simulink library "slx_LJM"  (R2024b)
settings: Solver=VariableStepAuto  StartTime=0.0  StopTime=10.0  RelTol=1e-3
libraries: simulink x3
settings Model: Creator=JulianBell  LastModifiedBy=GavinWilliamson
settings RTWCC: GPUComputeCapability=3.5

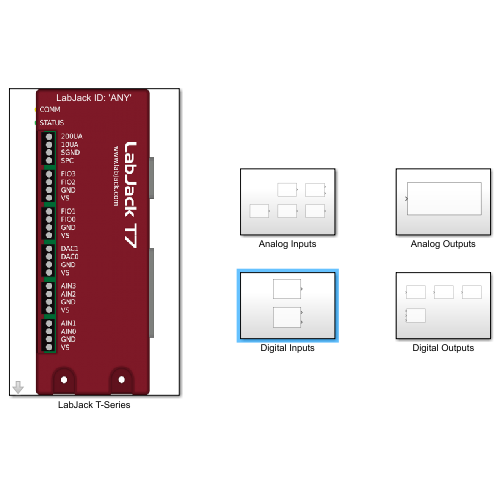
[thumbnail: Simulink's stored preview of the top-level diagram]
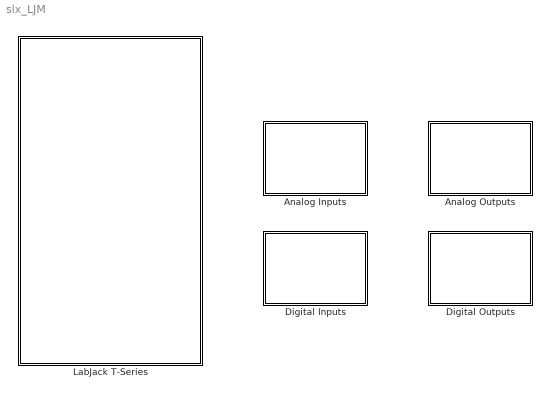
== system slx_LJM ==
  Analog Inputs : Subsystem
  Analog Outputs : Subsystem
  Digital Inputs : Subsystem
  Digital Outputs : Subsystem
  LabJack T-Series : Subsystem  mask{ljIdentifier='ANY', cnx_mth=USB, ljHandle=[]}
      mask prompts: ljIdentifier "LabJack Identifier [char]"; cnx_mth "Connection Method"; ljHandle "LabJack Handle"
      mask DialogControl DescGroupVar Prompt: LabJack T-Series
      mask DialogControl DescTextVar Prompt: This block is used to connect to a LabJack T4 or T7 device. Individual ports on the device can be configured, read, and written to by placing other blocks in the "slx_LJM" library within this block. This library link on this block must be disabled to place those block within this block.
      mask DialogControl Control4 Prompt: Once a simulation is stopped, the connection to the DIO ports are disabled, the LabJack clocks sare set to their default settings, and then the LabJack is disconnected. This is done through a Level-2 S-function block with the corresponding code in the "close_lbj.m" file.
      mask DialogControl Control2 Prompt: You can scan for any device that can be seen by inputting 'ANY' into the "LabJack Identifier" parameter. To connect to a specific device the serial number, IP address, or device name can be used. For more information please look at the documentaiton below.
      mask DialogControl Control3 Prompt: LabJack Connection Documentation
      mask Display:
      | image('ljT7.png');
      | idString = ["\color{White} LabJack ID: "+ get_param(gcb, 'ljIdentifier')];
      | text(0.5,0.98,idString,'horizontalAlignment','center','texmode','on');
      | 
      | %disp();

== system slx_LJM/Analog Inputs ==
  lj_AINRead : Subsystem  mask{ljPort="AIN0", ljRange=+/- 10V, Diff_Rd_SW=off, Diff_Rd="AIN1", ljHandle=32}
      mask prompts: ljPort "Port Name:"; ljRange "Voltage Range: (T7 Only)"; Diff_Rd_SW "Enable"; Diff_Rd "Negative Channel"; ljHandle "LabJack Handle"
      mask DialogControl DescGroupVar Prompt: AIN Read
      mask DialogControl DescTextVar Prompt: This block is used to read an analog input port. If using a T7 device the voltage range can be selected, and a differential reading can be chosen. If a differential reading is chosen, a valid negative channel must also be selected (typically the odd port for a pair of ports).  Voltage range selection and differential readings are not available on T4 devices.
      mask DialogControl Control4 Prompt: *For T4 devices the voltage range will be set to the default of the port (either +/- 10V or +/-2.5V) The parameter radio button do not effect the configuration.
      mask DialogControl Control3 Prompt: Differential Reading Documentation
      mask DialogControl Container3 Prompt: Differential Read (T7 Only)
      mask Display: disp(["AIN Read", "Port: "+ get_param(gcb, 'ljPort')]);
  lj_CurrentRead : Subsystem  mask{ljPort="AIN1", ljHandle=32, currentL=4, currentH=20, outputL=4, outputH=20}
      mask prompts: ljPort "Port Name:"; ljHandle "LabJack Handle"; currentL "Low Current (mA)"; currentH "High Current (mA)"; outputL "Low Output Value"; outputH "High Output Value"
      mask DialogControl DescGroupVar Prompt: Current Read
      mask DialogControl DescTextVar Prompt: This block is used for reading a current signal that is passed into the designated port using a LabJack current shunt. The block outputs the raw current reading as well as the scaled output based on the ranges set in the mask. The high and low output values correspond to the range of the sensor that you are reading.
      mask DialogControl Control2 Prompt: Current Shunt Documentation
      mask Display: disp(["Current Read", "Port: "+ get_param(gcb, 'ljPort')]);
  lj_RTDRead : Subsystem  mask{ljPort="AIN1", ljHandle=-1, rtdType=PT100, tempUnit=C, refResistance=1K}
      mask prompts: ljPort "Port Name:"; ljHandle "LabJack Handle"; rtdType "RTD Type"; tempUnit "Temperature Unit"; refResistance "Reference Resistance"
      mask DialogControl DescGroupVar Prompt: RTD Read
      mask DialogControl DescTextVar Prompt: This block is used to read an RTD.  The RTD type, temperature unit, and reference resistance can all be selected. This block assumes that exitation circuit #4 is being used, which is often implemented through the LabJack Resistance Tick.
      mask DialogControl RTD_doc Prompt: LabJack RTD Documentation
      mask DialogControl Ex_circ_4 Prompt: Excitation Circuit #4
      mask DialogControl res_tick Prompt: LabJack Resistance Tick
      mask Display: disp(["RTD Read", "Port: "+ get_param(gcb, 'ljPort')]);
  lj_ThermistorRead : Subsystem  mask{ljPort="AIN1", ljHandle=32, thermRes=1000, tempUnit=C, refResistance=10K, a=1.032e-3, b=2.387e-4, c=0, d=1.58e-7}
      mask prompts: ljPort "Port Name:"; ljHandle "LabJack Handle"; thermRes "Thermistor Resistance"; tempUnit "Temperature Unit"; refResistance "Reference Resistance"
      mask TypeOptions tempUnit: C | F | K
      mask DialogControl DescGroupVar Prompt: Thermistor Read
      mask DialogControl DescTextVar Prompt: This block is used to read a thermistor. This block assumes that exitation ciruit #4 is being used, which is often implemented thorugh a LabJack Resistance Tick. This block also configures the LabJack port to use the Steinhart-Hart equation. This configuartion can be altered in the mask's initialization code. The thermistor restistance, temperature unit, reference resistance, and Steinhart-Hart coefficients can all be set using the block's mask.
      mask DialogControl thermistor_doc Prompt: LabJack Thermistor Documentation
      mask DialogControl ex_circ_4 Prompt: Exitation Ciruit #4
      mask DialogControl res_tick Prompt: LabJack Resistance Tick
      mask DialogControl Container3 Prompt: Steinhart-Hart Coefficients
      mask Display: disp(["Thermistor Read", "Port: "+ get_param(gcb, 'ljPort')]);
  lj_ThermocoupleRead : Subsystem  mask{ljPort="AIN0", tempUnit=C, thermocoupleType=K, Diff_Rd_SW=off, Diff_Rd="AIN1", ljHandle=32}
      mask prompts: ljPort "Port Name:"; tempUnit "Temperature Units"; thermocoupleType "Thermocouple Type"; Diff_Rd_SW "Enable"; Diff_Rd "Negative Channel"; ljHandle "LabJack Handle"
      mask TypeOptions tempUnit: K | C | F
      mask TypeOptions thermocoupleType: E | J | K | R | T | S | N | B | C
      mask DialogControl DescGroupVar Prompt: Thermocouple Read
      mask DialogControl DescTextVar Prompt: This block is used to read a thermocouple. The thermocouple type and temperature units can be set in the block's mask. Differential reading can be enabled. If a differential reading is chosen, a valid negative channel must also be selected (typically the odd port for a pair of ports). This block only functions with T7 devices, not T4.
      mask DialogControl thermocouple_doc Prompt: LabJack Thermocouple Documentation
      mask DialogControl thermocouple_wir Prompt: LabJack Thermocouple Wiring
      mask DialogControl Container3 Prompt: Differential Read (T7 Only)
      mask Display: disp(["Thermocouple Read", "Port: "+ get_param(gcb, 'ljPort')]);

== system slx_LJM/Analog Outputs ==
  lj_DACWrite : Subsystem  mask{ljPort="DAC0", ljHandle=0}
      mask prompts: ljPort "LabJack DAC Port"; ljHandle "LabJack Handle"
      mask DialogControl DescGroupVar Prompt: DAC Write
      mask DialogControl DescTextVar Prompt: Block is used to output an analog signal throught the DAC ports. The typical output range for a T4/T7 device is 0-5V.
      mask DialogControl Control2 Prompt: LabJack DAC Documentation
      mask Display: disp(["DAC Write", "Port: "+ get_param(gcb, 'ljPort')]);

== system slx_LJM/Digital Inputs ==
  lj_DIORead : Subsystem  mask{ljPort="FIO1", ljHandle=[]}
      mask prompts: ljPort "Port ID"; ljHandle "LabJack Handle"
      mask DialogControl DescGroupVar Prompt: DIO Read
      mask DialogControl DescTextVar Prompt: This block is used to read a digital input port. An output value of 1 corresponds with a "high" value and an output value of 0 corresponds with a "low" value.
      mask DialogControl Control2 Prompt: LabJack Digital I/O Documentation
      mask Display: disp(["DIO Read", "Port: "+ get_param(gcb, 'ljPort')]);
  lj_FrequencyRead : Subsystem  mask{ljPort="DIO1", meas_typ=Rising-to-Rising Edge, ljClock=Clock 0 (32-bit), ljHandle=[]}
      mask prompts: ljPort "Port ID"; meas_typ "Measurement Type"; ljClock "Select LabJack Clock"; ljHandle "LabJack Handle"
      mask DialogControl DescGroupVar Prompt: Frequency Read
      mask DialogControl DescTextVar Prompt: This block is used to take a frequency reading of a diginal input port. The Port ID must be in the format "DIO#" so that the corresponding LabJack port can be properly configured. The measurement type and LabJack clock used to read frequency can also be selected. Caution should be used when selecting a LabJack clock to ensure there are no conflicts with other blocks in the LabJack. For more information, please see the documentation below.
      mask DialogControl Control2 Prompt: *It has been observed that the LabJack will occasionally read a period of 0 and a frequency of "nan" between valid reading of the correct frequency.
      mask DialogControl freq_in_data Prompt: LabJack Frequency In Datasheet
      mask DialogControl config_freq_in Prompt: Configuring & Reading Frequency
      mask DialogControl clock_web Prompt: LabJack Clock Source
      mask Display: disp(["Frequency Read", "Port: "+ get_param(gcb, 'ljPort')]);

== system slx_LJM/Digital Outputs ==
  lj_DACTickWrite : Subsystem  mask{ljPort="FIO0", ljHandle=2}
      mask prompts: ljPort "Port ID"; ljHandle "LabJack Handle"
      mask DialogControl DescGroupVar Prompt: DAC Tick Write
      mask DialogControl DescTextVar Prompt: This block is desinged to be used with a LabJack DAC to write a +/-10V signal out of a digital output port. This block will cause the LabJack matlab library to error if a DAC tick is not connected to the correct port.
      mask DialogControl Control2 Prompt: Labjack DAC Tick Documentation
      mask Display: disp(["DAC Tick Write", "Port: "+ get_param(gcb, 'ljPort')]);
  lj_DIOWrite : Subsystem  mask{ljPort="FIO0", defaultState=Low, ljHandle=2}
      mask prompts: ljPort "Port ID"; defaultState "Default Output State"; ljHandle "LabJack Handle"
      mask DialogControl DescGroupVar Prompt: DIO Write
      mask DialogControl DescTextVar Prompt: This block is used to write out of a digital output port. The default output state can be chosen. An input constant of 1 corresponds to a "high" value being written and an input constant of 0 corresponds with a "low" value being written.
      mask DialogControl Control2 Prompt: LabJack Digital I/O Documentation
      mask Display: disp(["DIO Write", "Port: "+ get_param(gcb, 'ljPort')]);
  lj_Heartbeat : Subsystem  mask{ljPort="FIO0", Simulink_step=1, ljHandle=2}
      mask prompts: ljPort "Port ID"; Simulink_step "Simulink Sample Time"; ljHandle "LabJack Handle"
      mask DialogControl DescGroupVar Prompt: Heartbeat
      mask DialogControl DescTextVar Prompt: This block is intended to be used as a watchdog to ensure that Simulink and the Labjack are still communicating properly. A 50% duty PWM is generated out of the specified port with the period that is passed into the input of the block. The sample time (step size) of the Simulink model must also be input into the mask parameters. The period input must be twice that of the Simulink sample time, and ideally 10x to ensure the most reliable performance of this block.
      mask Display: disp(["Heartbeat", "Port: "+ get_param(gcb, 'ljPort')]);
  lj_PWM : Subsystem  mask{ljPort="DIO0", defaultState=Low, ljClock=Clock 0 (32-bit), ljHandle=2}
      mask prompts: ljPort "Port ID"; defaultState "Default Output State"; ljClock "Select LabJack Clock"; ljHandle "LabJack Handle"
      mask DialogControl DescGroupVar Prompt: DIO PWM Write
      mask DialogControl DescTextVar Prompt: This block is used to write a PWM signal out of a DIO port. The portname should be in the format "DIO#" so that the port can be properly configured. The frequency, duty cycle, and enabling of the PWM is controlled by the block's input ports and can be updated while the simulatioin is running. A default output state can be chosen as well as the LabJack Clock that the PWM will use. Caution must be used when selecting which clock especially if multiple PWM write or read blocks are used in the same LabJack block. Please refer to the documentation below for addtional information.
      mask DialogControl pwm_data Prompt: LabJack PWM Out Datasheet
      mask DialogControl pwm_config Prompt: Configuring a PWM Output
      mask DialogControl clock_web Prompt: LabJack Clock Source
      mask Display: disp(["DIO PWM Write", "Port: "+ get_param(gcb, 'ljPort')]);

== system slx_LJM/LabJack T-Series ==
  Constant : Constant  Value=ljHandle
  Display : Display
  Level-2 MATLAB S-Function : M-S-Function  FunctionName=close_lbj
      mask DialogControl DescGroupVar Prompt: close_lbj
      mask DialogControl DescTextVar Prompt: Level 2 S-Function
      mask DialogControl Control2 Prompt: Block takes the input of the Labjack Handle as an int32 signal, and outputs the handle as a int 32 signal. Block closes connection to the LabJack when a simulation is stopped.
  wires:
  Constant/1 -> Level-2 MATLAB S-Function/1
  Level-2 MATLAB S-Function/1 -> Display/1

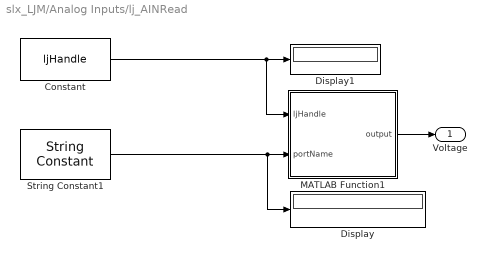
== system slx_LJM/Analog Inputs/lj_AINRead ==
  Constant : Constant  Value=ljHandle
  Display : Display
  Display1 : Display
  MATLAB Function1 : MATLAB Function  TreatAsAtomicUnit=on
  String Constant1 : StringConstant  String=ljPort
  Voltage : Outport
  wires:
  Constant/1 -> Display1/1, MATLAB Function1/1(ljHandle)
  MATLAB Function1/1(output) -> Voltage/1
  String Constant1/1 -> MATLAB Function1/2(portName), Display/1

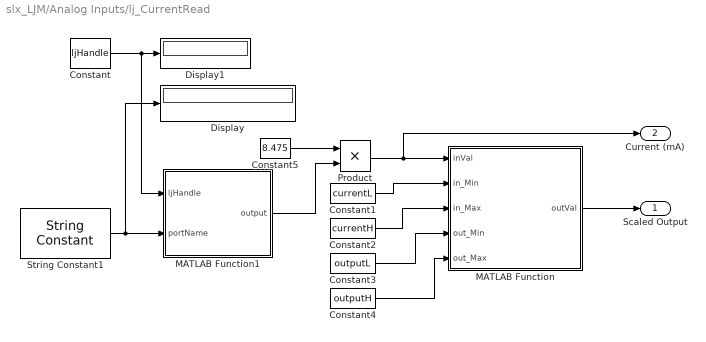
== system slx_LJM/Analog Inputs/lj_CurrentRead ==
  Constant : Constant  Value=ljHandle
  Constant1 : Constant  Value=currentL
  Constant2 : Constant  Value=currentH
  Constant3 : Constant  Value=outputL
  Constant4 : Constant  Value=outputH
  Constant5 : Constant  Value=8.475
  Display : Display
  Display1 : Display
  MATLAB Function : MATLAB Function  TreatAsAtomicUnit=on
  MATLAB Function1 : MATLAB Function  TreatAsAtomicUnit=on
  Product : Product
  String Constant1 : StringConstant  String=ljPort
  Scaled Output : Outport
  Current (mA) : Outport  Port=2
  wires:
  String Constant1/1 -> Display/1, MATLAB Function1/2(portName)
  Constant/1 -> MATLAB Function1/1(ljHandle), Display1/1
  Constant5/1 -> Product/1
  MATLAB Function1/1(output) -> Product/2
  Constant1/1 -> MATLAB Function/2(in_Min)
  Product/1 -> Current (mA)/1, MATLAB Function/1(inVal)
  Constant2/1 -> MATLAB Function/3(in_Max)
  Constant3/1 -> MATLAB Function/4(out_Min)
  Constant4/1 -> MATLAB Function/5(out_Max)
  MATLAB Function/1(outVal) -> Scaled Output/1

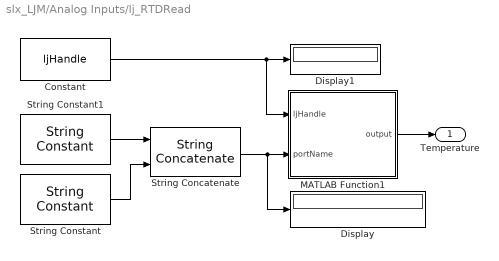
== system slx_LJM/Analog Inputs/lj_RTDRead ==
  Constant : Constant  Value=ljHandle
  Display : Display
  Display1 : Display
  MATLAB Function1 : MATLAB Function  TreatAsAtomicUnit=on
  String Concatenate : StringConcatenate
  String Constant : StringConstant  String='_EF_READ_A'
  String Constant1 : StringConstant  String=ljPort
  Temperature : Outport
  wires:
  String Constant1/1 -> String Concatenate/1
  Constant/1 -> Display1/1, MATLAB Function1/1(ljHandle)
  MATLAB Function1/1(output) -> Temperature/1
  String Constant/1 -> String Concatenate/2
  String Concatenate/1 -> MATLAB Function1/2(portName), Display/1

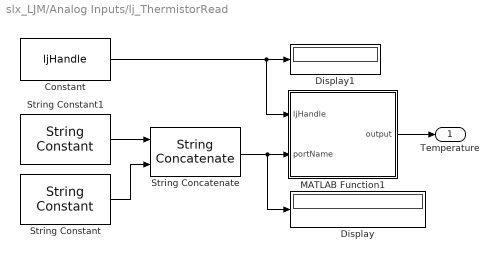
== system slx_LJM/Analog Inputs/lj_ThermistorRead ==
  Constant : Constant  Value=ljHandle
  Display : Display
  Display1 : Display
  MATLAB Function1 : MATLAB Function  TreatAsAtomicUnit=on
  String Concatenate : StringConcatenate
  String Constant : StringConstant  String='_EF_READ_A'
  String Constant1 : StringConstant  String=ljPort
  Temperature : Outport
  wires:
  String Concatenate/1 -> Display/1, MATLAB Function1/2(portName)
  String Constant/1 -> String Concatenate/2
  MATLAB Function1/1(output) -> Temperature/1
  Constant/1 -> MATLAB Function1/1(ljHandle), Display1/1
  String Constant1/1 -> String Concatenate/1

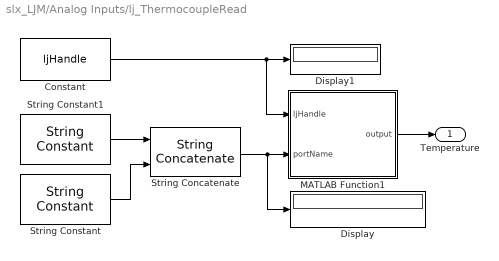
== system slx_LJM/Analog Inputs/lj_ThermocoupleRead ==
  Constant : Constant  Value=ljHandle
  Display : Display
  Display1 : Display
  MATLAB Function1 : MATLAB Function  TreatAsAtomicUnit=on
  String Concatenate : StringConcatenate
  String Constant : StringConstant  String='_EF_READ_A'
  String Constant1 : StringConstant  String=ljPort
  Temperature : Outport
  wires:
  String Constant1/1 -> String Concatenate/1
  Constant/1 -> Display1/1, MATLAB Function1/1(ljHandle)
  MATLAB Function1/1(output) -> Temperature/1
  String Constant/1 -> String Concatenate/2
  String Concatenate/1 -> MATLAB Function1/2(portName), Display/1

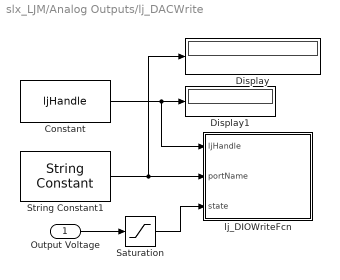
== system slx_LJM/Analog Outputs/lj_DACWrite ==
  Output Voltage : Inport
  Constant : Constant  Value=ljHandle
  Display : Display
  Display1 : Display
  Saturation : Saturate  UpperLimit=5  LowerLimit=0
  String Constant1 : StringConstant  String=ljPort
  lj_DIOWriteFcn : MATLAB Function  TreatAsAtomicUnit=on
  wires:
  Constant/1 -> lj_DIOWriteFcn/1(ljHandle), Display1/1
  Output Voltage/1 -> Saturation/1
  String Constant1/1 -> lj_DIOWriteFcn/2(portName), Display/1
  Saturation/1 -> lj_DIOWriteFcn/3(state)

== system slx_LJM/Digital Inputs/lj_DIORead ==
  Constant : Constant  Value=ljHandle
  Display : Display
  Display1 : Display
  MATLAB Function1 : MATLAB Function  TreatAsAtomicUnit=on
  String Constant1 : StringConstant  String=ljPort
  State : Outport
  wires:
  String Constant1/1 -> Display/1, MATLAB Function1/2(portName)
  MATLAB Function1/1(output) -> State/1
  Constant/1 -> MATLAB Function1/1(ljHandle), Display1/1

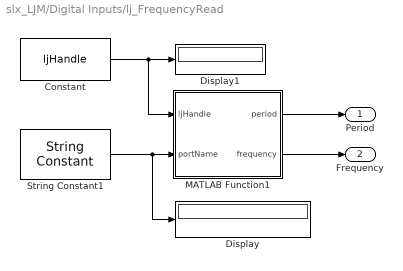
== system slx_LJM/Digital Inputs/lj_FrequencyRead ==
  Constant : Constant  Value=ljHandle
  Display : Display
  Display1 : Display
  MATLAB Function1 : MATLAB Function  TreatAsAtomicUnit=on
  String Constant1 : StringConstant  String=ljPort
  Period : Outport
  Frequency : Outport  Port=2
  wires:
  String Constant1/1 -> Display/1, MATLAB Function1/2(portName)
  Constant/1 -> MATLAB Function1/1(ljHandle), Display1/1
  MATLAB Function1/1(period) -> Period/1
  MATLAB Function1/2(frequency) -> Frequency/1

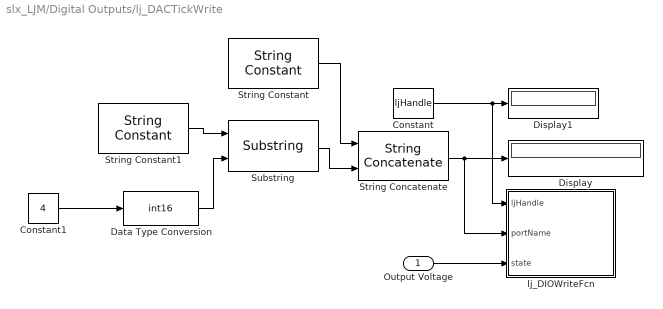
== system slx_LJM/Digital Outputs/lj_DACTickWrite ==
  Output Voltage : Inport
  Constant : Constant  Value=ljHandle
  Constant1 : Constant  Value=4
  Data Type Conversion : DataTypeConversion  OutDataTypeStr=int16  SaturateOnIntegerOverflow=off  RndMeth=Floor
  Display : Display
  Display1 : Display
  String Concatenate : StringConcatenate
  String Constant : StringConstant  String='TDAC'
  String Constant1 : StringConstant  String=ljPort
  Substring : Substring  StringFromIdxToEnd=on
  lj_DIOWriteFcn : MATLAB Function  TreatAsAtomicUnit=on
  wires:
  String Constant1/1 -> Substring/1
  Constant1/1 -> Data Type Conversion/1
  String Concatenate/1 -> Display/1, lj_DIOWriteFcn/2(portName)
  Substring/1 -> String Concatenate/2
  String Constant/1 -> String Concatenate/1
  Constant/1 -> Display1/1, lj_DIOWriteFcn/1(ljHandle)
  Output Voltage/1 -> lj_DIOWriteFcn/3(state)
  Data Type Conversion/1 -> Substring/2

== system slx_LJM/Digital Outputs/lj_DIOWrite ==
  State : Inport
  Constant : Constant  Value=ljHandle
  Display : Display
  Display1 : Display
  String Constant1 : StringConstant  String=ljPort
  lj_DIOWriteFcn : MATLAB Function  TreatAsAtomicUnit=on
  wires:
  String Constant1/1 -> lj_DIOWriteFcn/2(portName), Display/1
  Constant/1 -> lj_DIOWriteFcn/1(ljHandle), Display1/1
  State/1 -> lj_DIOWriteFcn/3(state)

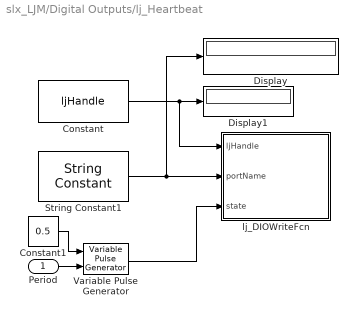
== system slx_LJM/Digital Outputs/lj_Heartbeat ==
  Period : Inport
  Constant : Constant  Value=ljHandle
  Constant1 : Constant  Value=0.5
  Display : Display
  Display1 : Display
  String Constant1 : StringConstant  String=ljPort
  Variable Pulse Generator : VariablePulseGenerator  RunAtFixedTimeIntervals=on  SampleTime=Simulink_step
  lj_DIOWriteFcn : MATLAB Function  TreatAsAtomicUnit=on
  wires:
  String Constant1/1 -> lj_DIOWriteFcn/2(portName), Display/1
  Constant/1 -> lj_DIOWriteFcn/1(ljHandle), Display1/1
  Variable Pulse Generator/1 -> lj_DIOWriteFcn/3(state)
  Period/1 -> Variable Pulse Generator/2
  Constant1/1 -> Variable Pulse Generator/1

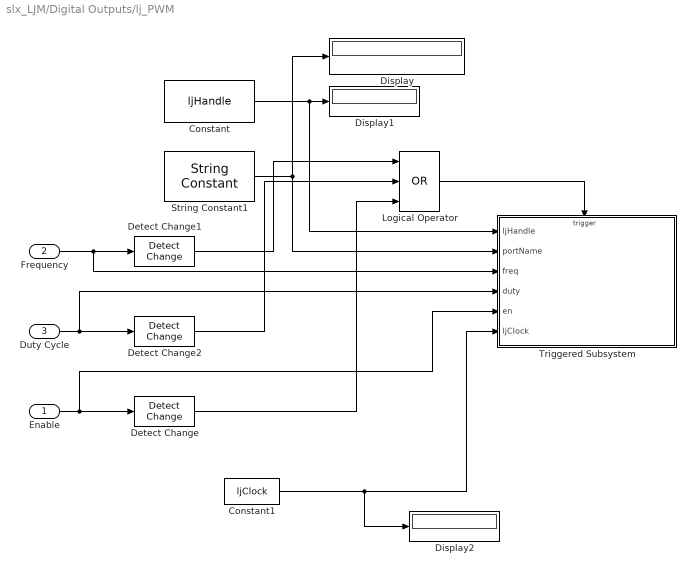
== system slx_LJM/Digital Outputs/lj_PWM ==
  Enable : Inport
  Frequency : Inport  Port=2
  Duty Cycle : Inport  Port=3
  Constant : Constant  Value=ljHandle
  Constant1 : Constant  Value=ljClock
  Detect Change : simulink/Logic and Bit Operations/Detect Change  vinit=0  OutDataTypeStr=boolean
  Detect Change1 : simulink/Logic and Bit Operations/Detect Change  vinit=0  OutDataTypeStr=boolean
  Detect Change2 : simulink/Logic and Bit Operations/Detect Change  vinit=0  OutDataTypeStr=boolean
  Display : Display
  Display1 : Display
  Display2 : Display
  Logical Operator : Logic  Operator=OR  Inputs=3  AllPortsSameDT=off  OutDataTypeStr=boolean
  String Constant1 : StringConstant  String=ljPort
  Triggered Subsystem : Subsystem  TreatAsAtomicUnit=on
  wires:
  String Constant1/1 -> Display/1, Triggered Subsystem/2(portName)
  Constant/1 -> Triggered Subsystem/1(ljHandle), Display1/1
  Enable/1 -> Triggered Subsystem/5(en), Detect Change/1
  Duty Cycle/1 -> Triggered Subsystem/4(duty), Detect Change2/1
  Frequency/1 -> Triggered Subsystem/3(freq), Detect Change1/1
  Logical Operator/1 -> Triggered Subsystem/Trigger
  Detect Change1/1 -> Logical Operator/1
  Detect Change2/1 -> Logical Operator/2
  Detect Change/1 -> Logical Operator/3
  Constant1/1 -> Display2/1, Triggered Subsystem/6(ljClock)

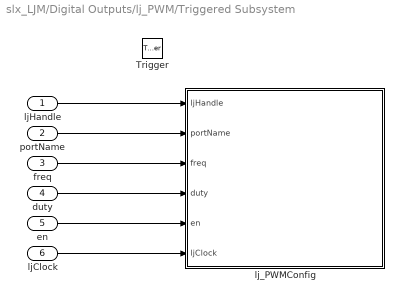
== system slx_LJM/Digital Outputs/lj_PWM/Triggered Subsystem ==
  ljHandle : Inport
  portName : Inport  Port=2
  freq : Inport  Port=3
  duty : Inport  Port=4
  en : Inport  Port=5
  ljClock : Inport  Port=6
  Trigger : TriggerPort  VariantControl=(inherit)  InitialTriggerSignalState=zero
  lj_PWMConfig : MATLAB Function  TreatAsAtomicUnit=on
  wires:
  ljHandle/1 -> lj_PWMConfig/1(ljHandle)
  portName/1 -> lj_PWMConfig/2(portName)
  freq/1 -> lj_PWMConfig/3(freq)
  duty/1 -> lj_PWMConfig/4(duty)
  en/1 -> lj_PWMConfig/5(en)
  ljClock/1 -> lj_PWMConfig/6(ljClock)

== matlab function slx_LJM/Digital Inputs/lj_FrequencyRead/MATLAB Function1 ==
  data: ljHandle input; portName input; period output; frequency output
function [period, frequency]  = fcn(ljHandle, portName)
coder.extrinsic('slx_eReadName')
period = [0];
frequency = [0];
portName_per = portName + "_EF_READ_A_F"
portName_freq = portName + "_EF_READ_B_F"
portName_reset = portName + "_EF_READ_A_F_AND_RESET"
%[~, period] = slx_eReadName(ljHandle, portName_per)
%[~, frequency] = slx_eReadName(ljHandle, portName_freq)
[~, period] = slx_eReadName(ljHandle, portName_reset)

frequency = 1/period;

== matlab function slx_LJM/Digital Outputs/lj_PWM/Triggered Subsystem/lj_PWMConfig ==
  data: ljHandle input; portName input; freq input; duty input; en input; ljClock input
function fcn(ljHandle,portName, freq, duty, en, ljClock)
coder.extrinsic('slx_eWriteName');
coder.extrinsic('slx_eReadName');

%set up addresses for configuring port
ljClock_str = string(ljClock);
addr1 = portName + "_EF_ENABLE";
addr2 = "DIO_EF_CLOCK" + ljClock_str + "_ENABLE";
addr3 = "DIO_EF_CLOCK" + ljClock_str + "_ROLL_VALUE";
addr4 = portName + "_EF_INDEX";
addr5 = portName + "_EF_CONFIG_A";
addr6 = portName + "_EF_CLOCK_SOURCE";

%disable channel and clock for configuration
if ljClock ~=0
    slx_eWriteName(ljHandle, "DIO_EF_CLOCK0_ENABLE",0)
else 
    slx_eWriteName(ljHandle, "DIO_EF_CLOCK1_ENABLE",0)
    slx_eWriteName(ljHandle, "DIO_EF_CLOCK2_ENABLE",0)
end
slx_eWriteName(ljHandle,addr1, 0);
slx_eWriteName(ljHandle,addr2, 0);
slx_eReadName(ljHandle,portName)

roll = round((80* 10^6)/freq); %valid for T4/T7 with 80MHz clock
Config_A = round((duty/100)*roll);

%configure PWM
slx_eWriteName(ljHandle,addr3, roll);
slx_eWriteName(ljHandle, addr6, ljClock);
slx_eWriteName(ljHandle,addr4, 0);
slx_eWriteName(ljHandle,addr5, Config_A);

%enable PWM
slx_eWriteName(ljHandle,addr2, 1);
slx_eWriteName(ljHandle,addr1, en);

end

== matlab function slx_LJM/Digital Outputs/lj_Heartbeat/lj_DIOWriteFcn ==
  data: ljHandle input; portName input; state input
function fcn(ljHandle,portName, state)
coder.extrinsic('slx_eWriteName')
slx_eWriteName(ljHandle, portName, state);

== matlab function slx_LJM/Analog Inputs/lj_ThermistorRead/MATLAB Function1 ==
  data: ljHandle input; portName input; output output
function output  = fcn(ljHandle, portName)
coder.extrinsic('slx_eReadName')
output = [0];
[~, output] = slx_eReadName(ljHandle, portName);

== matlab function slx_LJM/Analog Inputs/lj_AINRead/MATLAB Function1 ==
  data: ljHandle input; portName input; output output
function output  = fcn(ljHandle, portName)
coder.extrinsic('slx_eReadName')
output = [0];
[~, output] = slx_eReadName(ljHandle, portName);

== matlab function slx_LJM/Analog Inputs/lj_ThermocoupleRead/MATLAB Function1 ==
  data: ljHandle input; portName input; output output
function output  = fcn(ljHandle, portName)
coder.extrinsic('slx_eReadName')
output = [0];
[~, output] = slx_eReadName(ljHandle, portName);

== matlab function slx_LJM/Analog Inputs/lj_RTDRead/MATLAB Function1 ==
  data: ljHandle input; portName input; output output
function output  = fcn(ljHandle, portName)
coder.extrinsic('slx_eReadName')
output = [0];
[~, output] = slx_eReadName(ljHandle, portName);

== matlab function slx_LJM/Digital Inputs/lj_DIORead/MATLAB Function1 ==
  data: ljHandle input; portName input; output output
function output  = fcn(ljHandle, portName)
coder.extrinsic('slx_eReadName')
output = [0];
[~, output] = slx_eReadName(ljHandle, portName);

== matlab function slx_LJM/Digital Outputs/lj_DIOWrite/lj_DIOWriteFcn ==
  data: ljHandle input; portName input; state input
function fcn(ljHandle,portName, state)
coder.extrinsic('slx_eWriteName')
slx_eWriteName(ljHandle, portName, state);

== matlab function slx_LJM/Digital Outputs/lj_DACTickWrite/lj_DIOWriteFcn ==
  data: ljHandle input; portName input; state input
function fcn(ljHandle,portName, state)
coder.extrinsic('slx_eWriteName')
slx_eWriteName(ljHandle, portName, state);

== matlab function slx_LJM/Analog Inputs/lj_CurrentRead/MATLAB Function1 ==
  data: ljHandle input; portName input; output output
function output  = fcn(ljHandle, portName)
coder.extrinsic('slx_eReadName')
output = [0];
[~, output] = slx_eReadName(ljHandle, portName);

== matlab function slx_LJM/Analog Inputs/lj_CurrentRead/MATLAB Function ==
  data: inVal input; outVal output; in_Min input; in_Max input; out_Min input; out_Max input
function outVal  = maprange(inVal,in_Min,in_Max,out_Min,out_Max)
%MAPRANGE Matlab implementation of simple Arduino maprange function
%   Source: https://www.arduino.cc/reference/en/language/functions/math/map/
outVal = (inVal - in_Min) * (out_Max - out_Min)/(in_Max - in_Min) + out_Min;
end

== matlab function slx_LJM/Analog Outputs/lj_DACWrite/lj_DIOWriteFcn ==
  data: ljHandle input; portName input; state input
function fcn(ljHandle,portName, state)
coder.extrinsic('slx_eWriteName')
slx_eWriteName(ljHandle, portName, state);
